simulink model "balance_leg"  (R2022b)
settings: Solver=VariableStepAuto  StartTime=0.0  StopTime=9  RelTol=1e-3
values from neighbouring files (symbols this model uses):
  K = get_K_from_LQR(R_w,R_l,l_l,l_r,l_wl,l_wr,l_bl,l_br,l_c,m_w,m_l,m_b,I_w,I_ll,I_lr,I_b,I_z,g,              R_w_ac,R_l_ac,l_l_ac,l_r_ac,l_wl_ac,l_wr_ac,l_bl_ac,l_br_ac,              l_c_ac,m_w_ac,m_l_ac,m_b_ac,I_w_ac,I_ll_ac,I_lr_ac,I_b_ac,I_z_ac,g_ac,              A,B,lqr_Q,lqr_R)    [HerKules_VOCAL_SJ_LQR_v4_with_data.m]    (also in HerKules_legth_K.m = lqr(A_num, B_num, lqr_Q, lqr_R); get_legth_k.m = lqr(JA,JB,Q,R); lqr_k.m = reshape([mt1,mt2,mt3,mt4,mt5,mt6,mt7,mt8,mt9,mt10,mt11,mt12]; niheK.m = sym('K',[2 6]))
  N = NM + mp*diff(x + L*sin(theta),t,2)    [get_legth_k.m]    (also in niheK.m)
undefined symbols (not defined in the file or in its folder): X, Y, Z
libraries: sm_lib x56, nesl_utility x22, slpidlib x2
(part 3 of 3)

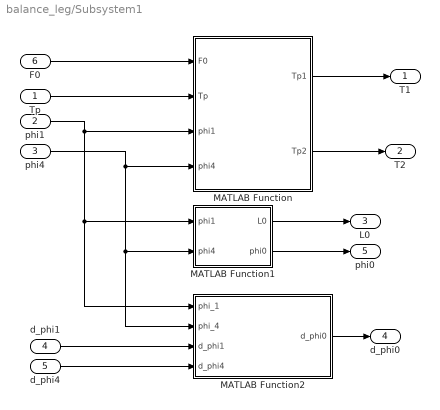
== system balance_leg/Subsystem1 ==
  Tp : Inport
  phi1 : Inport  Port=2
  phi4 : Inport  Port=3
  d_phi1 : Inport  Port=4
  d_phi4 : Inport  Port=5
  F0 : Inport  Port=6
  MATLAB Function : MATLAB Function  TreatAsAtomicUnit=on
  MATLAB Function1 : MATLAB Function  TreatAsAtomicUnit=on
  MATLAB Function2 : MATLAB Function  TreatAsAtomicUnit=on
  T1 : Outport
  T2 : Outport  Port=2
  L0 : Outport  Port=3
  d_phi0 : Outport  Port=4
  phi0 : Outport  Port=5
  wires:
  F0/1 -> MATLAB Function/1(F0)
  Tp/1 -> MATLAB Function/2(Tp)
  phi1/1 -> MATLAB Function2/1(phi_1), MATLAB Function1/1(phi1), MATLAB Function/3(phi1)
  phi4/1 -> MATLAB Function2/2(phi_4), MATLAB Function1/2(phi4), MATLAB Function/4(phi4)
  d_phi4/1 -> MATLAB Function2/4(d_phi4)
  d_phi1/1 -> MATLAB Function2/3(d_phi1)
  MATLAB Function/1(Tp1) -> T1/1
  MATLAB Function/2(Tp2) -> T2/1
  MATLAB Function1/1(L0) -> L0/1
  MATLAB Function1/2(phi0) -> phi0/1
  MATLAB Function2/1(d_phi0) -> d_phi0/1

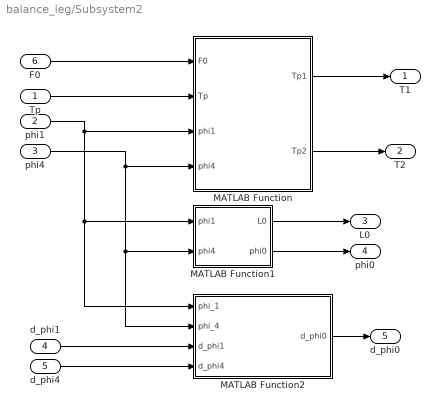
== system balance_leg/Subsystem2 ==
  Tp : Inport
  phi1 : Inport  Port=2
  phi4 : Inport  Port=3
  d_phi1 : Inport  Port=4
  d_phi4 : Inport  Port=5
  F0 : Inport  Port=6
  MATLAB Function : MATLAB Function  TreatAsAtomicUnit=on
  MATLAB Function1 : MATLAB Function  TreatAsAtomicUnit=on
  MATLAB Function2 : MATLAB Function  TreatAsAtomicUnit=on
  T1 : Outport
  T2 : Outport  Port=2
  L0 : Outport  Port=3
  phi0 : Outport  Port=4
  d_phi0 : Outport  Port=5
  wires:
  F0/1 -> MATLAB Function/1(F0)
  Tp/1 -> MATLAB Function/2(Tp)
  phi1/1 -> MATLAB Function2/1(phi_1), MATLAB Function1/1(phi1), MATLAB Function/3(phi1)
  phi4/1 -> MATLAB Function2/2(phi_4), MATLAB Function1/2(phi4), MATLAB Function/4(phi4)
  d_phi4/1 -> MATLAB Function2/4(d_phi4)
  d_phi1/1 -> MATLAB Function2/3(d_phi1)
  MATLAB Function/1(Tp1) -> T1/1
  MATLAB Function/2(Tp2) -> T2/1
  MATLAB Function1/1(L0) -> L0/1
  MATLAB Function1/2(phi0) -> phi0/1
  MATLAB Function2/1(d_phi0) -> d_phi0/1

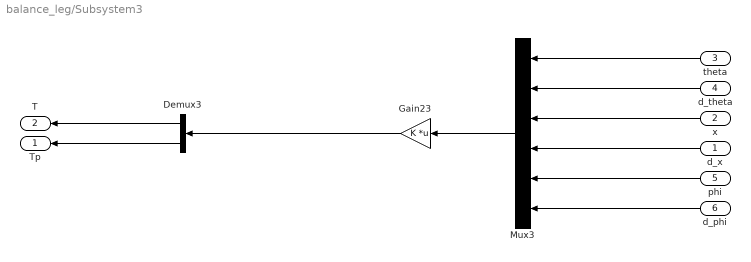
== system balance_leg/Subsystem3 ==
  d_x : Inport
  x : Inport  Port=2
  theta : Inport  Port=3
  d_theta : Inport  Port=4
  phi : Inport  Port=5
  d_phi : Inport  Port=6
  Demux3 : Demux  Outputs=2
  Gain23 : Gain  Gain=K  Multiplication=Matrix(K*u) (u vector)
  Mux3 : Mux  Inputs=6
  Tp : Outport
  T : Outport  Port=2
  wires:
  d_phi/1 -> Mux3/6
  Demux3/1 -> T/1
  d_theta/1 -> Mux3/2
  Mux3/1 -> Gain23/1
  Gain23/1 -> Demux3/1
  phi/1 -> Mux3/5
  x/1 -> Mux3/3
  theta/1 -> Mux3/1
  Demux3/2 -> Tp/1
  d_x/1 -> Mux3/4

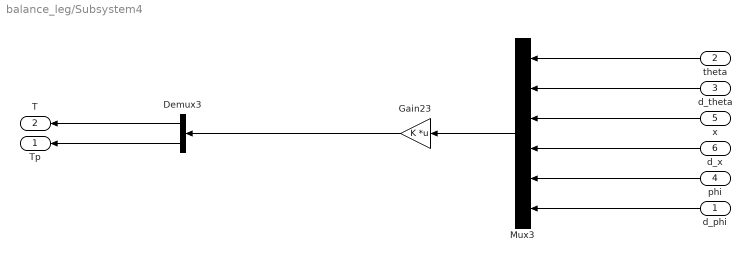
== system balance_leg/Subsystem4 ==
  d_phi : Inport
  theta : Inport  Port=2
  d_theta : Inport  Port=3
  phi : Inport  Port=4
  x : Inport  Port=5
  d_x : Inport  Port=6
  Demux3 : Demux  Outputs=2
  Gain23 : Gain  Gain=K  Multiplication=Matrix(K*u) (u vector)
  Mux3 : Mux  Inputs=6
  Tp : Outport
  T : Outport  Port=2
  wires:
  d_phi/1 -> Mux3/6
  Demux3/1 -> T/1
  d_theta/1 -> Mux3/2
  Mux3/1 -> Gain23/1
  Gain23/1 -> Demux3/1
  phi/1 -> Mux3/5
  x/1 -> Mux3/3
  theta/1 -> Mux3/1
  Demux3/2 -> Tp/1
  d_x/1 -> Mux3/4

== matlab function balance_leg/Subsystem1/MATLAB Function ==
  data: F0 input; Tp1 output; Tp input; phi1 input; phi4 input; Tp2 output
function [Tp1,Tp2] = VM_cal(F0,Tp,phi1,phi4)
% syms T1 T2 F0 Tp phi1 phi4 XE l1 l2 l3 l4
l5=0.15;
l1=0.15;
l2=0.27;
l3=0.27;
l4=0.15;

YD = l4*sin(phi4);
YB = l1*sin(phi1);
XD = l5 + l4*cos(phi4);
XB = l1*cos(phi1); 
lBD = sqrt((XD - XB)*(XD - XB) + (YD - YB)*(YD - YB));
A0 = 2*l2*(XD - XB);
B0 = 2*l2*(YD - YB);
C0 = l2*l2 + lBD*lBD - l3*l3;
phi2 = 2*atan2((B0 + sqrt(A0*A0 + B0*B0 - C0*C0)),A0 + C0);
phi3 = atan2(YB-YD+l2*sin(phi2),XB-XD+l2*cos(phi2));
XC = l1*cos(phi1) + l2*cos(phi2);
YC = l1*sin(phi1) + l2*sin(phi2);
L0 = sqrt((XC - l5/2)*(XC - l5/2) + YC*YC);
phi0 = atan2(YC,XC - l5/2);
j11 = (l1*sin(phi0-phi3)*sin(phi1-phi2))/sin(phi3-phi2);
j12 = (l1*cos(phi0-phi3)*sin(phi1-phi2))/L0*sin(phi3-phi2);
j21 = (l4*sin(phi0-phi2)*sin(phi3-phi4))/sin(phi3-phi2);
j22 = (l4*cos(phi0-phi2)*sin(phi3-phi4))/L0*sin(phi3-phi2);
J = [j11 j12; j21 j22];
F = [F0;Tp];
T = J * F;
Tp1 = T(1,1);
Tp2 = T(2,1);
end

== matlab function balance_leg/Subsystem1/MATLAB Function1 ==
  data: phi1 input; L0 output; phi4 input; phi0 output
function [L0,phi0] = get_legparam(phi1,phi4)
    l5=0.15;
    l1=0.15;
    l2=0.27;
    l3=0.27;
    l4=0.15;
    YD = l4*sin(phi4);
    YB = l1*sin(phi1);
    XD = l5 + l4*cos(phi4);
    XB = l1*cos(phi1); 
    lBD = sqrt((XD - XB)*(XD - XB) + (YD - YB)*(YD - YB));
    A0 = 2*l2*(XD - XB);
    B0 = 2*l2*(YD - YB);
    C0 = l2*l2 + lBD*lBD - l3*l3;
    phi2 = 2*atan2((B0 + sqrt(A0*A0 + B0*B0 - C0*C0)),(A0 + C0));
    XC = l1*cos(phi1) + l2*cos(phi2);
    YC = l1*sin(phi1) + l2*sin(phi2);
    L0 = sqrt((XC - l5/2)*(XC - l5/2) + YC*YC);
    phi0=atan2(YC,(XC-l5/2));
end

== matlab function balance_leg/Subsystem1/MATLAB Function2 ==
  data: phi_1 input; d_phi0 output; phi_4 input; d_phi1 input; d_phi4 input
function d_phi0 = get_dphi0(phi_1,phi_4,d_phi1,d_phi4)
    l5=0.15;
    l1=0.15;
    l2=0.27;
    l3=0.27;
    l4=0.15;
    d_phi0 = (d_phi1*((l1*cos(phi_1) + (2*l2*cos(2*atan(((4*l2^2*(l1*sin(phi_1) - l4*sin(phi_4))^2 - ((l1*sin(phi_1) - l4*sin(phi_4))^2 + (l5 - l1*cos(phi_1) + l4*cos(phi_4))^2 + l2^2 - l3^2)^2 + 4*l2^2*(l5 - l1*cos(phi_1) + l4*cos(phi_4))^2)^(1/2) - 2*l2*(l1*sin(phi_1) - l4*sin(phi_4)))/((l1*sin(phi_1) - l4*sin(phi_4))^2 + (l5 - l1*cos(phi_1) + l4*cos(phi_4))^2 + l2^2 - l3^2 + 2*l2*(l5 - l1*cos(phi_1) + l4*cos(phi_4)))))*(((8*l1*l2^2*cos(phi_1)*(l1*sin(phi_1) - l4*sin(phi_4)) - 2*(2*l1*cos(phi_1)*(l1*sin(phi_1) - l4*sin(phi_4)) + 2*l1*sin(phi_1)*(l5 - l1*cos(phi_1) + l4*cos(phi_4)))*((l1*sin(phi_1) - l4*sin(phi_4))^2 + (l5 - l1*cos(phi_1) + l4*cos(phi_4))^2 + l2^2 - l3^2) + 8*l1*l2^2*sin(phi_1)*(l5 - l1*cos(phi_1) + l4*cos(phi_4)))/(2*(4*l2^2*(l1*sin(phi_1) - l4*sin(phi_4))^2 - ((l1*sin(phi_1) - l4*sin(phi_4))^2 + (l5 - l1*cos(phi_1) + l4*cos(phi_4))^2 + l2^2 - l3^2)^2 + 4*l2^2*(l5 - l1*cos(phi_1) + l4*cos(phi_4))^2)^(1/2)) - 2*l1*l2*cos(phi_1))/((l1*sin(phi_1) - l4*sin(phi_4))^2 + (l5 - l1*cos(phi_1) + l4*cos(phi_4))^2 + l2^2 - l3^2 + 2*l2*(l5 - l1*cos(phi_1) + l4*cos(phi_4))) - (((4*l2^2*(l1*sin(phi_1) - l4*sin(phi_4))^2 - ((l1*sin(phi_1) - l4*sin(phi_4))^2 + (l5 - l1*cos(phi_1) + l4*cos(phi_4))^2 + l2^2 - l3^2)^2 + 4*l2^2*(l5 - l1*cos(phi_1) + l4*cos(phi_4))^2)^(1/2) - 2*l2*(l1*sin(phi_1) - l4*sin(phi_4)))*(2*l1*l2*sin(phi_1) + 2*l1*cos(phi_1)*(l1*sin(phi_1) - l4*sin(phi_4)) + 2*l1*sin(phi_1)*(l5 - l1*cos(phi_1) + l4*cos(phi_4))))/((l1*sin(phi_1) - l4*sin(phi_4))^2 + (l5 - l1*cos(phi_1) + l4*cos(phi_4))^2 + l2^2 - l3^2 + 2*l2*(l5 - l1*cos(phi_1) + l4*cos(phi_4)))^2))/(((4*l2^2*(l1*sin(phi_1) - l4*sin(phi_4))^2 - ((l1*sin(phi_1) - l4*sin(phi_4))^2 + (l5 - l1*cos(phi_1) + l4*cos(phi_4))^2 + l2^2 - l3^2)^2 + 4*l2^2*(l5 - l1*cos(phi_1) + l4*cos(phi_4))^2)^(1/2) - 2*l2*(l1*sin(phi_1) - l4*sin(phi_4)))^2/((l1*sin(phi_1) - l4*sin(phi_4))^2 + (l5 - l1*cos(phi_1) + l4*cos(phi_4))^2 + l2^2 - l3^2 + 2*l2*(l5 - l1*cos(phi_1) + l4*cos(phi_4)))^2 + 1))/(l2*cos(2*atan(((4*l2^2*(l1*sin(phi_1) - l4*sin(phi_4))^2 - ((l1*sin(phi_1) - l4*sin(phi_4))^2 + (l5 - l1*cos(phi_1) + l4*cos(phi_4))^2 + l2^2 - l3^2)^2 + 4*l2^2*(l5 - l1*cos(phi_1) + l4*cos(phi_4))^2)^(1/2) - 2*l2*(l1*sin(phi_1) - l4*sin(phi_4)))/((l1*sin(phi_1) - l4*sin(phi_4))^2 + (l5 - l1*cos(phi_1) + l4*cos(phi_4))^2 + l2^2 - l3^2 + 2*l2*(l5 - l1*cos(phi_1) + l4*cos(phi_4))))) - l5/2 + l1*cos(phi_1)) + ((l2*sin(2*atan(((4*l2^2*(l1*sin(phi_1) - l4*sin(phi_4))^2 - ((l1*sin(phi_1) - l4*sin(phi_4))^2 + (l5 - l1*cos(phi_1) + l4*cos(phi_4))^2 + l2^2 - l3^2)^2 + 4*l2^2*(l5 - l1*cos(phi_1) + l4*cos(phi_4))^2)^(1/2) - 2*l2*(l1*sin(phi_1) - l4*sin(phi_4)))/((l1*sin(phi_1) - l4*sin(phi_4))^2 + (l5 - l1*cos(phi_1) + l4*cos(phi_4))^2 + l2^2 - l3^2 + 2*l2*(l5 - l1*cos(phi_1) + l4*cos(phi_4))))) + l1*sin(phi_1))*(l1*sin(phi_1) + (2*l2*sin(2*atan(((4*l2^2*(l1*sin(phi_1) - l4*sin(phi_4))^2 - ((l1*sin(phi_1) - l4*sin(phi_4))^2 + (l5 - l1*cos(phi_1) + l4*cos(phi_4))^2 + l2^2 - l3^2)^2 + 4*l2^2*(l5 - l1*cos(phi_1) + l4*cos(phi_4))^2)^(1/2) - 2*l2*(l1*sin(phi_1) - l4*sin(phi_4)))/((l1*sin(phi_1) - l4*sin(phi_4))^2 + (l5 - l1*cos(phi_1) + l4*cos(phi_4))^2 + l2^2 - l3^2 + 2*l2*(l5 - l1*cos(phi_1) + l4*cos(phi_4)))))*(((8*l1*l2^2*cos(phi_1)*(l1*sin(phi_1) - l4*sin(phi_4)) - 2*(2*l1*cos(phi_1)*(l1*sin(phi_1) - l4*sin(phi_4)) + 2*l1*sin(phi_1)*(l5 - l1*cos(phi_1) + l4*cos(phi_4)))*((l1*sin(phi_1) - l4*sin(phi_4))^2 + (l5 - l1*cos(phi_1) + l4*cos(phi_4))^2 + l2^2 - l3^2) + 8*l1*l2^2*sin(phi_1)*(l5 - l1*cos(phi_1) + l4*cos(phi_4)))/(2*(4*l2^2*(l1*sin(phi_1) - l4*sin(phi_4))^2 - ((l1*sin(phi_1) - l4*sin(phi_4))^2 + (l5 - l1*cos(phi_1) + l4*cos(phi_4))^2 + l2^2 - l3^2)^2 + 4*l2^2*(l5 - l1*cos(phi_1) + l4*cos(phi_4))^2)^(1/2)) - 2*l1*l2*cos(phi_1))/((l1*sin(phi_1) - l4*sin(phi_4))^2 + (l5 - l1*cos(phi_1) + l4*cos(phi_4))^2 + l2^2 - l3^2 + 2*l2*(l5 - l1*cos(phi_1) + l4*cos(phi_4))) - (((4*l2^2*(l1*sin(phi_1) - l4*sin(phi_4))^2 - ((l1*sin(phi_1) - l4*sin(phi_4))^2 + (l5 - l1*cos(phi_1) + l4*cos(phi_4))^2 + l2^2 - l3^2)^2 + 4*l2^2*(l5 - l1*cos(phi_1) + l4*cos(phi_4))^2)^(1/2) - 2*l2*(l1*sin(phi_1) - l4*sin(phi_4)))*(2*l1*l2*sin(phi_1) + 2*l1*cos(phi_1)*(l1*sin(phi_1) - l4*sin(phi_4)) + 2*l1*sin(phi_1)*(l5 - l1*cos(phi_1) + l4*cos(phi_4))))/((l1*sin(phi_1) - l4*sin(phi_4))^2 + (l5 - l1*cos(phi_1) + l4*cos(phi_4))^2 + l2^2 - l3^2 + 2*l2*(l5 - l1*cos(phi_1) + l4*cos(phi_4)))^2))/(((4*l2^2*(l1*sin(phi_1) - l4*sin(phi_4))^2 - ((l1*sin(phi_1) - l4*sin(phi_4))^2 + (l5 - l1*cos(phi_1) + l4*cos(phi_4))^2 + l2^2 - l3^2)^2 + 4*l2^2*(l5 - l1*cos(phi_1) + l4*cos(phi_4))^2)^(1/2) - 2*l2*(l1*sin(phi_1) - l4*sin(phi_4)))^2/((l1*sin(phi_1) - l4*sin(phi_4))^2 + (l5 - l1*cos(phi_1) + l4*cos(phi_4))^2 + l2^2 - l3^2 + 2*l2*(l5 - l1*cos(phi_1) + l4*cos(phi_4)))^2 + 1)))/(l2*cos(2*atan(((4*l2^2*(l1*sin(phi_1) - l4*sin(phi_4))^2 - ((l1*sin(phi_1) - l4*sin(phi_4))^2 + (l5 - l1*cos(phi_1) + l4*cos(phi_4))^2 + l2^2 - l3^2)^2 + 4*l2^2*(l5 - l1*cos(phi_1) + l4*cos(phi_4))^2)^(1/2) - 2*l2*(l1*sin(phi_1) - l4*sin(phi_4)))/((l1*sin(phi_1) - l4*sin(phi_4))^2 + (l5 - l1*cos(phi_1) + l4*cos(phi_4))^2 + l2^2 - l3^2 + 2*l2*(l5 - l1*cos(phi_1) + l4*cos(phi_4))))) - l5/2 + l1*cos(phi_1))^2))/((l2*sin(2*atan(((4*l2^2*(l1*sin(phi_1) - l4*sin(phi_4))^2 - ((l1*sin(phi_1) - l4*sin(phi_4))^2 + (l5 - l1*cos(phi_1) + l4*cos(phi_4))^2 + l2^2 - l3^2)^2 + 4*l2^2*(l5 - l1*cos(phi_1) + l4*cos(phi_4))^2)^(1/2) - 2*l2*(l1*sin(phi_1) - l4*sin(phi_4)))/((l1*sin(phi_1) - l4*sin(phi_4))^2 + (l5 - l1*cos(phi_1) + l4*cos(phi_4))^2 + l2^2 - l3^2 + 2*l2*(l5 - l1*cos(phi_1) + l4*cos(phi_4))))) + l1*sin(phi_1))^2/(l2*cos(2*atan(((4*l2^2*(l1*sin(phi_1) - l4*sin(phi_4))^2 - ((l1*sin(phi_1) - l4*sin(phi_4))^2 + (l5 - l1*cos(phi_1) + l4*cos(phi_4))^2 + l2^2 - l3^2)^2 + 4*l2^2*(l5 - l1*cos(phi_1) + l4*cos(phi_4))^2)^(1/2) - 2*l2*(l1*sin(phi_1) - l4*sin(phi_4)))/((l1*sin(phi_1) - l4*sin(phi_4))^2 + (l5 - l1*cos(phi_1) + l4*cos(phi_4))^2 + l2^2 - l3^2 + 2*l2*(l5 - l1*cos(phi_1) + l4*cos(phi_4))))) - l5/2 + l1*cos(phi_1))^2 + 1) - (d_phi4*((2*l2*cos(2*atan(((4*l2^2*(l1*sin(phi_1) - l4*sin(phi_4))^2 - ((l1*sin(phi_1) - l4*sin(phi_4))^2 + (l5 - l1*cos(phi_1) + l4*cos(phi_4))^2 + l2^2 - l3^2)^2 + 4*l2^2*(l5 - l1*cos(phi_1) + l4*cos(phi_4))^2)^(1/2) - 2*l2*(l1*sin(phi_1) - l4*sin(phi_4)))/((l1*sin(phi_1) - l4*sin(phi_4))^2 + (l5 - l1*cos(phi_1) + l4*cos(phi_4))^2 + l2^2 - l3^2 + 2*l2*(l5 - l1*cos(phi_1) + l4*cos(phi_4)))))*(((8*l2^2*l4*cos(phi_4)*(l1*sin(phi_1) - l4*sin(phi_4)) - 2*(2*l4*cos(phi_4)*(l1*sin(phi_1) - l4*sin(phi_4)) + 2*l4*sin(phi_4)*(l5 - l1*cos(phi_1) + l4*cos(phi_4)))*((l1*sin(phi_1) - l4*sin(phi_4))^2 + (l5 - l1*cos(phi_1) + l4*cos(phi_4))^2 + l2^2 - l3^2) + 8*l2^2*l4*sin(phi_4)*(l5 - l1*cos(phi_1) + l4*cos(phi_4)))/(2*(4*l2^2*(l1*sin(phi_1) - l4*sin(phi_4))^2 - ((l1*sin(phi_1) - l4*sin(phi_4))^2 + (l5 - l1*cos(phi_1) + l4*cos(phi_4))^2 + l2^2 - l3^2)^2 + 4*l2^2*(l5 - l1*cos(phi_1) + l4*cos(phi_4))^2)^(1/2)) - 2*l2*l4*cos(phi_4))/((l1*sin(phi_1) - l4*sin(phi_4))^2 + (l5 - l1*cos(phi_1) + l4*cos(phi_4))^2 + l2^2 - l3^2 + 2*l2*(l5 - l1*cos(phi_1) + l4*cos(phi_4))) - (((4*l2^2*(l1*sin(phi_1) - l4*sin(phi_4))^2 - ((l1*sin(phi_1) - l4*sin(phi_4))^2 + (l5 - l1*cos(phi_1) + l4*cos(phi_4))^2 + l2^2 - l3^2)^2 + 4*l2^2*(l5 - l1*cos(phi_1) + l4*cos(phi_4))^2)^(1/2) - 2*l2*(l1*sin(phi_1) - l4*sin(phi_4)))*(2*l2*l4*sin(phi_4) + 2*l4*cos(phi_4)*(l1*sin(phi_1) - l4*sin(phi_4)) + 2*l4*sin(phi_4)*(l5 - l1*cos(phi_1) + l4*cos(phi_4))))/((l1*sin(phi_1) - l4*sin(phi_4))^2 + (l5 - l1*cos(phi_1) + l4*cos(phi_4))^2 + l2^2 - l3^2 + 2*l2*(l5 - l1*cos(phi_1) + l4*cos(phi_4)))^2))/((((4*l2^2*(l1*sin(phi_1) - l4*sin(phi_4))^2 - ((l1*sin(phi_1) - l4*sin(phi_4))^2 + (l5 - l1*cos(phi_1) + l4*cos(phi_4))^2 + l2^2 - l3^2)^2 + 4*l2^2*(l5 - l1*cos(phi_1) + l4*cos(phi_4))^2)^(1/2) - 2*l2*(l1*sin(phi_1) - l4*sin(phi_4)))^2/((l1*sin(phi_1) - l4*sin(phi_4))^2 + (l5 - l1*cos(phi_1) + l4*cos(phi_4))^2 + l2^2 - l3^2 + 2*l2*(l5 - l1*cos(phi_1) + l4*cos(phi_4)))^2 + 1)*(l2*cos(2*atan(((4*l2^2*(l1*sin(phi_1) - l4*sin(phi_4))^2 - ((l1*sin(phi_1) - l4*sin(phi_4))^2 + (l5 - l1*cos(phi_1) + l4*cos(phi_4))^2 + l2^2 - l3^2)^2 + 4*l2^2*(l5 - l1*cos(phi_1) + l4*cos(phi_4))^2)^(1/2) - 2*l2*(l1*sin(phi_1) - l4*sin(phi_4)))/((l1*sin(phi_1) - l4*sin(phi_4))^2 + (l5 - l1*cos(phi_1) + l4*cos(phi_4))^2 + l2^2 - l3^2 + 2*l2*(l5 - l1*cos(phi_1) + l4*cos(phi_4))))) - l5/2 + l1*cos(phi_1))) + (2*l2*sin(2*atan(((4*l2^2*(l1*sin(phi_1) - l4*sin(phi_4))^2 - ((l1*sin(phi_1) - l4*sin(phi_4))^2 + (l5 - l1*cos(phi_1) + l4*cos(phi_4))^2 + l2^2 - l3^2)^2 + 4*l2^2*(l5 - l1*cos(phi_1) + l4*cos(phi_4))^2)^(1/2) - 2*l2*(l1*sin(phi_1) - l4*sin(phi_4)))/((l1*sin(phi_1) - l4*sin(phi_4))^2 + (l5 - l1*cos(phi_1) + l4*cos(phi_4))^2 + l2^2 - l3^2 + 2*l2*(l5 - l1*cos(phi_1) + l4*cos(phi_4)))))*(l2*sin(2*atan(((4*l2^2*(l1*sin(phi_1) - l4*sin(phi_4))^2 - ((l1*sin(phi_1) - l4*sin(phi_4))^2 + (l5 - l1*cos(phi_1) + l4*cos(phi_4))^2 + l2^2 - l3^2)^2 + 4*l2^2*(l5 - l1*cos(phi_1) + l4*cos(phi_4))^2)^(1/2) - 2*l2*(l1*sin(phi_1) - l4*sin(phi_4)))/((l1*sin(phi_1) - l4*sin(phi_4))^2 + (l5 - l1*cos(phi_1) + l4*cos(phi_4))^2 + l2^2 - l3^2 + 2*l2*(l5 - l1*cos(phi_1) + l4*cos(phi_4))))) + l1*sin(phi_1))*(((8*l2^2*l4*cos(phi_4)*(l1*sin(phi_1) - l4*sin(phi_4)) - 2*(2*l4*cos(phi_4)*(l1*sin(phi_1) - l4*sin(phi_4)) + 2*l4*sin(phi_4)*(l5 - l1*cos(phi_1) + l4*cos(phi_4)))*((l1*sin(phi_1) - l4*sin(phi_4))^2 + (l5 - l1*cos(phi_1) + l4*cos(phi_4))^2 + l2^2 - l3^2) + 8*l2^2*l4*sin(phi_4)*(l5 - l1*cos(phi_1) + l4*cos(phi_4)))/(2*(4*l2^2*(l1*sin(phi_1) - l4*sin(phi_4))^2 - ((l1*sin(phi_1) - l4*sin(phi_4))^2 + (l5 - l1*cos(phi_1) + l4*cos(phi_4))^2 + l2^2 - l3^2)^2 + 4*l2^2*(l5 - l1*cos(phi_1) + l4*cos(phi_4))^2)^(1/2)) - 2*l2*l4*cos(phi_4))/((l1*sin(phi_1) - l4*sin(phi_4))^2 + (l5 - l1*cos(phi_1) + l4*cos(phi_4))^2 + l2^2 - l3^2 + 2*l2*(l5 - l1*cos(phi_1) + l4*cos(phi_4))) - (((4*l2^2*(l1*sin(phi_1) - l4*sin(phi_4))^2 - ((l1*sin(phi_1) - l4*sin(phi_4))^2 + (l5 - l1*cos(phi_1) + l4*cos(phi_4))^2 + l2^2 - l3^2)^2 + 4*l2^2*(l5 - l1*cos(phi_1) + l4*cos(phi_4))^2)^(1/2) - 2*l2*(l1*sin(phi_1) - l4*sin(phi_4)))*(2*l2*l4*sin(phi_4) + 2*l4*cos(phi_4)*(l1*sin(phi_1) - l4*sin(phi_4)) + 2*l4*sin(phi_4)*(l5 - l1*cos(phi_1) + l4*cos(phi_4))))/((l1*sin(phi_1) - l4*sin(phi_4))^2 + (l5 - l1*cos(phi_1) + l4*cos(phi_4))^2 + l2^2 - l3^2 + 2*l2*(l5 - l1*cos(phi_1) + l4*cos(phi_4)))^2))/((((4*l2^2*(l1*sin(phi_1) - l4*sin(phi_4))^2 - ((l1*sin(phi_1) - l4*sin(phi_4))^2 + (l5 - l1*cos(phi_1) + l4*cos(phi_4))^2 + l2^2 - l3^2)^2 + 4*l2^2*(l5 - l1*cos(phi_1) + l4*cos(phi_4))^2)^(1/2) - 2*l2*(l1*sin(phi_1) - l4*sin(phi_4)))^2/((l1*sin(phi_1) - l4*sin(phi_4))^2 + (l5 - l1*cos(phi_1) + l4*cos(phi_4))^2 + l2^2 - l3^2 + 2*l2*(l5 - l1*cos(phi_1) + l4*cos(phi_4)))^2 + 1)*(l2*cos(2*atan(((4*l2^2*(l1*sin(phi_1) - l4*sin(phi_4))^2 - ((l1*sin(phi_1) - l4*sin(phi_4))^2 + (l5 - l1*cos(phi_1) + l4*cos(phi_4))^2 + l2^2 - l3^2)^2 + 4*l2^2*(l5 - l1*cos(phi_1) + l4*cos(phi_4))^2)^(1/2) - 2*l2*(l1*sin(phi_1) - l4*sin(phi_4)))/((l1*sin(phi_1) - l4*sin(phi_4))^2 + (l5 - l1*cos(phi_1) + l4*cos(phi_4))^2 + l2^2 - l3^2 + 2*l2*(l5 - l1*cos(phi_1) + l4*cos(phi_4))))) - l5/2 + l1*cos(phi_1))^2)))/((l2*sin(2*atan(((4*l2^2*(l1*sin(phi_1) - l4*sin(phi_4))^2 - ((l1*sin(phi_1) - l4*sin(phi_4))^2 + (l5 - l1*cos(phi_1) + l4*cos(phi_4))^2 + l2^2 - l3^2)^2 + 4*l2^2*(l5 - l1*cos(phi_1) + l4*cos(phi_4))^2)^(1/2) - 2*l2*(l1*sin(phi_1) - l4*sin(phi_4)))/((l1*sin(phi_1) - l4*sin(phi_4))^2 + (l5 - l1*cos(phi_1) + l4*cos(phi_4))^2 + l2^2 - l3^2 + 2*l2*(l5 - l1*cos(phi_1) + l4*cos(phi_4))))) + l1*sin(phi_1))^2/(l2*cos(2*atan(((4*l2^2*(l1*sin(phi_1) - l4*sin(phi_4))^2 - ((l1*sin(phi_1) - l4*sin(phi_4))^2 + (l5 - l1*cos(phi_1) + l4*cos(phi_4))^2 + l2^2 - l3^2)^2 + 4*l2^2*(l5 - l1*cos(phi_1) + l4*cos(phi_4))^2)^(1/2) - 2*l2*(l1*sin(phi_1) - l4*sin(phi_4)))/((l1*sin(phi_1) - l4*sin(phi_4))^2 + (l5 - l1*cos(phi_1) + l4*cos(phi_4))^2 + l2^2 - l3^2 + 2*l2*(l5 - l1*cos(phi_1) + l4*cos(phi_4))))) - l5/2 + l1*cos(phi_1))^2 + 1);
end

== matlab function balance_leg/Subsystem2/MATLAB Function ==
  data: F0 input; Tp1 output; Tp input; phi1 input; phi4 input; Tp2 output
function [Tp1,Tp2] = VM_cal(F0,Tp,phi1,phi4)
% syms T1 T2 F0 Tp phi1 phi4 XE l1 l2 l3 l4
l5=0.15;
l1=0.15;
l2=0.27;
l3=0.27;
l4=0.15;

YD = l4*sin(phi4);
YB = l1*sin(phi1);
XD = l5 + l4*cos(phi4);
XB = l1*cos(phi1); 
lBD = sqrt((XD - XB)*(XD - XB) + (YD - YB)*(YD - YB));
A0 = 2*l2*(XD - XB);
B0 = 2*l2*(YD - YB);
C0 = l2*l2 + lBD*lBD - l3*l3;
phi2 = 2*atan2((B0 + sqrt(A0*A0 + B0*B0 - C0*C0)),A0 + C0);
phi3 = atan2(YB-YD+l2*sin(phi2),XB-XD+l2*cos(phi2));
XC = l1*cos(phi1) + l2*cos(phi2);
YC = l1*sin(phi1) + l2*sin(phi2);
L0 = sqrt((XC - l5/2)*(XC - l5/2) + YC*YC);
phi0 = atan2(YC,XC - l5/2);
j11 = (l1*sin(phi0-phi3)*sin(phi1-phi2))/sin(phi3-phi2);
j12 = (l1*cos(phi0-phi3)*sin(phi1-phi2))/L0*sin(phi3-phi2);
j21 = (l4*sin(phi0-phi2)*sin(phi3-phi4))/sin(phi3-phi2);
j22 = (l4*cos(phi0-phi2)*sin(phi3-phi4))/L0*sin(phi3-phi2);
J = [j11 j12; j21 j22];
F = [F0;Tp];
T = J * F;
Tp1 = T(1,1);
Tp2 = T(2,1);
end

== matlab function balance_leg/Subsystem2/MATLAB Function1 ==
  data: phi1 input; L0 output; phi4 input; phi0 output
function [L0,phi0] = get_legparam(phi1,phi4)
    l5=0.15;
    l1=0.15;
    l2=0.27;
    l3=0.27;
    l4=0.15;
    YD = l4*sin(phi4);
    YB = l1*sin(phi1);
    XD = l5 + l4*cos(phi4);
    XB = l1*cos(phi1); 
    lBD = sqrt((XD - XB)*(XD - XB) + (YD - YB)*(YD - YB));
    A0 = 2*l2*(XD - XB);
    B0 = 2*l2*(YD - YB);
    C0 = l2*l2 + lBD*lBD - l3*l3;
    phi2 = 2*atan2((B0 + sqrt(A0*A0 + B0*B0 - C0*C0)),(A0 + C0));
    XC = l1*cos(phi1) + l2*cos(phi2);
    YC = l1*sin(phi1) + l2*sin(phi2);
    L0 = sqrt((XC - l5/2)*(XC - l5/2) + YC*YC);
    phi0=atan2(YC,(XC-l5/2));
end

== matlab function balance_leg/Subsystem2/MATLAB Function2 ==
  data: phi_1 input; d_phi0 output; phi_4 input; d_phi1 input; d_phi4 input
function d_phi0 = get_dphi0(phi_1,phi_4,d_phi1,d_phi4)
    l5=0.15;
    l1=0.15;
    l2=0.27;
    l3=0.27;
    l4=0.15;
    d_phi0 = (d_phi1*((l1*cos(phi_1) + (2*l2*cos(2*atan(((4*l2^2*(l1*sin(phi_1) - l4*sin(phi_4))^2 - ((l1*sin(phi_1) - l4*sin(phi_4))^2 + (l5 - l1*cos(phi_1) + l4*cos(phi_4))^2 + l2^2 - l3^2)^2 + 4*l2^2*(l5 - l1*cos(phi_1) + l4*cos(phi_4))^2)^(1/2) - 2*l2*(l1*sin(phi_1) - l4*sin(phi_4)))/((l1*sin(phi_1) - l4*sin(phi_4))^2 + (l5 - l1*cos(phi_1) + l4*cos(phi_4))^2 + l2^2 - l3^2 + 2*l2*(l5 - l1*cos(phi_1) + l4*cos(phi_4)))))*(((8*l1*l2^2*cos(phi_1)*(l1*sin(phi_1) - l4*sin(phi_4)) - 2*(2*l1*cos(phi_1)*(l1*sin(phi_1) - l4*sin(phi_4)) + 2*l1*sin(phi_1)*(l5 - l1*cos(phi_1) + l4*cos(phi_4)))*((l1*sin(phi_1) - l4*sin(phi_4))^2 + (l5 - l1*cos(phi_1) + l4*cos(phi_4))^2 + l2^2 - l3^2) + 8*l1*l2^2*sin(phi_1)*(l5 - l1*cos(phi_1) + l4*cos(phi_4)))/(2*(4*l2^2*(l1*sin(phi_1) - l4*sin(phi_4))^2 - ((l1*sin(phi_1) - l4*sin(phi_4))^2 + (l5 - l1*cos(phi_1) + l4*cos(phi_4))^2 + l2^2 - l3^2)^2 + 4*l2^2*(l5 - l1*cos(phi_1) + l4*cos(phi_4))^2)^(1/2)) - 2*l1*l2*cos(phi_1))/((l1*sin(phi_1) - l4*sin(phi_4))^2 + (l5 - l1*cos(phi_1) + l4*cos(phi_4))^2 + l2^2 - l3^2 + 2*l2*(l5 - l1*cos(phi_1) + l4*cos(phi_4))) - (((4*l2^2*(l1*sin(phi_1) - l4*sin(phi_4))^2 - ((l1*sin(phi_1) - l4*sin(phi_4))^2 + (l5 - l1*cos(phi_1) + l4*cos(phi_4))^2 + l2^2 - l3^2)^2 + 4*l2^2*(l5 - l1*cos(phi_1) + l4*cos(phi_4))^2)^(1/2) - 2*l2*(l1*sin(phi_1) - l4*sin(phi_4)))*(2*l1*l2*sin(phi_1) + 2*l1*cos(phi_1)*(l1*sin(phi_1) - l4*sin(phi_4)) + 2*l1*sin(phi_1)*(l5 - l1*cos(phi_1) + l4*cos(phi_4))))/((l1*sin(phi_1) - l4*sin(phi_4))^2 + (l5 - l1*cos(phi_1) + l4*cos(phi_4))^2 + l2^2 - l3^2 + 2*l2*(l5 - l1*cos(phi_1) + l4*cos(phi_4)))^2))/(((4*l2^2*(l1*sin(phi_1) - l4*sin(phi_4))^2 - ((l1*sin(phi_1) - l4*sin(phi_4))^2 + (l5 - l1*cos(phi_1) + l4*cos(phi_4))^2 + l2^2 - l3^2)^2 + 4*l2^2*(l5 - l1*cos(phi_1) + l4*cos(phi_4))^2)^(1/2) - 2*l2*(l1*sin(phi_1) - l4*sin(phi_4)))^2/((l1*sin(phi_1) - l4*sin(phi_4))^2 + (l5 - l1*cos(phi_1) + l4*cos(phi_4))^2 + l2^2 - l3^2 + 2*l2*(l5 - l1*cos(phi_1) + l4*cos(phi_4)))^2 + 1))/(l2*cos(2*atan(((4*l2^2*(l1*sin(phi_1) - l4*sin(phi_4))^2 - ((l1*sin(phi_1) - l4*sin(phi_4))^2 + (l5 - l1*cos(phi_1) + l4*cos(phi_4))^2 + l2^2 - l3^2)^2 + 4*l2^2*(l5 - l1*cos(phi_1) + l4*cos(phi_4))^2)^(1/2) - 2*l2*(l1*sin(phi_1) - l4*sin(phi_4)))/((l1*sin(phi_1) - l4*sin(phi_4))^2 + (l5 - l1*cos(phi_1) + l4*cos(phi_4))^2 + l2^2 - l3^2 + 2*l2*(l5 - l1*cos(phi_1) + l4*cos(phi_4))))) - l5/2 + l1*cos(phi_1)) + ((l2*sin(2*atan(((4*l2^2*(l1*sin(phi_1) - l4*sin(phi_4))^2 - ((l1*sin(phi_1) - l4*sin(phi_4))^2 + (l5 - l1*cos(phi_1) + l4*cos(phi_4))^2 + l2^2 - l3^2)^2 + 4*l2^2*(l5 - l1*cos(phi_1) + l4*cos(phi_4))^2)^(1/2) - 2*l2*(l1*sin(phi_1) - l4*sin(phi_4)))/((l1*sin(phi_1) - l4*sin(phi_4))^2 + (l5 - l1*cos(phi_1) + l4*cos(phi_4))^2 + l2^2 - l3^2 + 2*l2*(l5 - l1*cos(phi_1) + l4*cos(phi_4))))) + l1*sin(phi_1))*(l1*sin(phi_1) + (2*l2*sin(2*atan(((4*l2^2*(l1*sin(phi_1) - l4*sin(phi_4))^2 - ((l1*sin(phi_1) - l4*sin(phi_4))^2 + (l5 - l1*cos(phi_1) + l4*cos(phi_4))^2 + l2^2 - l3^2)^2 + 4*l2^2*(l5 - l1*cos(phi_1) + l4*cos(phi_4))^2)^(1/2) - 2*l2*(l1*sin(phi_1) - l4*sin(phi_4)))/((l1*sin(phi_1) - l4*sin(phi_4))^2 + (l5 - l1*cos(phi_1) + l4*cos(phi_4))^2 + l2^2 - l3^2 + 2*l2*(l5 - l1*cos(phi_1) + l4*cos(phi_4)))))*(((8*l1*l2^2*cos(phi_1)*(l1*sin(phi_1) - l4*sin(phi_4)) - 2*(2*l1*cos(phi_1)*(l1*sin(phi_1) - l4*sin(phi_4)) + 2*l1*sin(phi_1)*(l5 - l1*cos(phi_1) + l4*cos(phi_4)))*((l1*sin(phi_1) - l4*sin(phi_4))^2 + (l5 - l1*cos(phi_1) + l4*cos(phi_4))^2 + l2^2 - l3^2) + 8*l1*l2^2*sin(phi_1)*(l5 - l1*cos(phi_1) + l4*cos(phi_4)))/(2*(4*l2^2*(l1*sin(phi_1) - l4*sin(phi_4))^2 - ((l1*sin(phi_1) - l4*sin(phi_4))^2 + (l5 - l1*cos(phi_1) + l4*cos(phi_4))^2 + l2^2 - l3^2)^2 + 4*l2^2*(l5 - l1*cos(phi_1) + l4*cos(phi_4))^2)^(1/2)) - 2*l1*l2*cos(phi_1))/((l1*sin(phi_1) - l4*sin(phi_4))^2 + (l5 - l1*cos(phi_1) + l4*cos(phi_4))^2 + l2^2 - l3^2 + 2*l2*(l5 - l1*cos(phi_1) + l4*cos(phi_4))) - (((4*l2^2*(l1*sin(phi_1) - l4*sin(phi_4))^2 - ((l1*sin(phi_1) - l4*sin(phi_4))^2 + (l5 - l1*cos(phi_1) + l4*cos(phi_4))^2 + l2^2 - l3^2)^2 + 4*l2^2*(l5 - l1*cos(phi_1) + l4*cos(phi_4))^2)^(1/2) - 2*l2*(l1*sin(phi_1) - l4*sin(phi_4)))*(2*l1*l2*sin(phi_1) + 2*l1*cos(phi_1)*(l1*sin(phi_1) - l4*sin(phi_4)) + 2*l1*sin(phi_1)*(l5 - l1*cos(phi_1) + l4*cos(phi_4))))/((l1*sin(phi_1) - l4*sin(phi_4))^2 + (l5 - l1*cos(phi_1) + l4*cos(phi_4))^2 + l2^2 - l3^2 + 2*l2*(l5 - l1*cos(phi_1) + l4*cos(phi_4)))^2))/(((4*l2^2*(l1*sin(phi_1) - l4*sin(phi_4))^2 - ((l1*sin(phi_1) - l4*sin(phi_4))^2 + (l5 - l1*cos(phi_1) + l4*cos(phi_4))^2 + l2^2 - l3^2)^2 + 4*l2^2*(l5 - l1*cos(phi_1) + l4*cos(phi_4))^2)^(1/2) - 2*l2*(l1*sin(phi_1) - l4*sin(phi_4)))^2/((l1*sin(phi_1) - l4*sin(phi_4))^2 + (l5 - l1*cos(phi_1) + l4*cos(phi_4))^2 + l2^2 - l3^2 + 2*l2*(l5 - l1*cos(phi_1) + l4*cos(phi_4)))^2 + 1)))/(l2*cos(2*atan(((4*l2^2*(l1*sin(phi_1) - l4*sin(phi_4))^2 - ((l1*sin(phi_1) - l4*sin(phi_4))^2 + (l5 - l1*cos(phi_1) + l4*cos(phi_4))^2 + l2^2 - l3^2)^2 + 4*l2^2*(l5 - l1*cos(phi_1) + l4*cos(phi_4))^2)^(1/2) - 2*l2*(l1*sin(phi_1) - l4*sin(phi_4)))/((l1*sin(phi_1) - l4*sin(phi_4))^2 + (l5 - l1*cos(phi_1) + l4*cos(phi_4))^2 + l2^2 - l3^2 + 2*l2*(l5 - l1*cos(phi_1) + l4*cos(phi_4))))) - l5/2 + l1*cos(phi_1))^2))/((l2*sin(2*atan(((4*l2^2*(l1*sin(phi_1) - l4*sin(phi_4))^2 - ((l1*sin(phi_1) - l4*sin(phi_4))^2 + (l5 - l1*cos(phi_1) + l4*cos(phi_4))^2 + l2^2 - l3^2)^2 + 4*l2^2*(l5 - l1*cos(phi_1) + l4*cos(phi_4))^2)^(1/2) - 2*l2*(l1*sin(phi_1) - l4*sin(phi_4)))/((l1*sin(phi_1) - l4*sin(phi_4))^2 + (l5 - l1*cos(phi_1) + l4*cos(phi_4))^2 + l2^2 - l3^2 + 2*l2*(l5 - l1*cos(phi_1) + l4*cos(phi_4))))) + l1*sin(phi_1))^2/(l2*cos(2*atan(((4*l2^2*(l1*sin(phi_1) - l4*sin(phi_4))^2 - ((l1*sin(phi_1) - l4*sin(phi_4))^2 + (l5 - l1*cos(phi_1) + l4*cos(phi_4))^2 + l2^2 - l3^2)^2 + 4*l2^2*(l5 - l1*cos(phi_1) + l4*cos(phi_4))^2)^(1/2) - 2*l2*(l1*sin(phi_1) - l4*sin(phi_4)))/((l1*sin(phi_1) - l4*sin(phi_4))^2 + (l5 - l1*cos(phi_1) + l4*cos(phi_4))^2 + l2^2 - l3^2 + 2*l2*(l5 - l1*cos(phi_1) + l4*cos(phi_4))))) - l5/2 + l1*cos(phi_1))^2 + 1) - (d_phi4*((2*l2*cos(2*atan(((4*l2^2*(l1*sin(phi_1) - l4*sin(phi_4))^2 - ((l1*sin(phi_1) - l4*sin(phi_4))^2 + (l5 - l1*cos(phi_1) + l4*cos(phi_4))^2 + l2^2 - l3^2)^2 + 4*l2^2*(l5 - l1*cos(phi_1) + l4*cos(phi_4))^2)^(1/2) - 2*l2*(l1*sin(phi_1) - l4*sin(phi_4)))/((l1*sin(phi_1) - l4*sin(phi_4))^2 + (l5 - l1*cos(phi_1) + l4*cos(phi_4))^2 + l2^2 - l3^2 + 2*l2*(l5 - l1*cos(phi_1) + l4*cos(phi_4)))))*(((8*l2^2*l4*cos(phi_4)*(l1*sin(phi_1) - l4*sin(phi_4)) - 2*(2*l4*cos(phi_4)*(l1*sin(phi_1) - l4*sin(phi_4)) + 2*l4*sin(phi_4)*(l5 - l1*cos(phi_1) + l4*cos(phi_4)))*((l1*sin(phi_1) - l4*sin(phi_4))^2 + (l5 - l1*cos(phi_1) + l4*cos(phi_4))^2 + l2^2 - l3^2) + 8*l2^2*l4*sin(phi_4)*(l5 - l1*cos(phi_1) + l4*cos(phi_4)))/(2*(4*l2^2*(l1*sin(phi_1) - l4*sin(phi_4))^2 - ((l1*sin(phi_1) - l4*sin(phi_4))^2 + (l5 - l1*cos(phi_1) + l4*cos(phi_4))^2 + l2^2 - l3^2)^2 + 4*l2^2*(l5 - l1*cos(phi_1) + l4*cos(phi_4))^2)^(1/2)) - 2*l2*l4*cos(phi_4))/((l1*sin(phi_1) - l4*sin(phi_4))^2 + (l5 - l1*cos(phi_1) + l4*cos(phi_4))^2 + l2^2 - l3^2 + 2*l2*(l5 - l1*cos(phi_1) + l4*cos(phi_4))) - (((4*l2^2*(l1*sin(phi_1) - l4*sin(phi_4))^2 - ((l1*sin(phi_1) - l4*sin(phi_4))^2 + (l5 - l1*cos(phi_1) + l4*cos(phi_4))^2 + l2^2 - l3^2)^2 + 4*l2^2*(l5 - l1*cos(phi_1) + l4*cos(phi_4))^2)^(1/2) - 2*l2*(l1*sin(phi_1) - l4*sin(phi_4)))*(2*l2*l4*sin(phi_4) + 2*l4*cos(phi_4)*(l1*sin(phi_1) - l4*sin(phi_4)) + 2*l4*sin(phi_4)*(l5 - l1*cos(phi_1) + l4*cos(phi_4))))/((l1*sin(phi_1) - l4*sin(phi_4))^2 + (l5 - l1*cos(phi_1) + l4*cos(phi_4))^2 + l2^2 - l3^2 + 2*l2*(l5 - l1*cos(phi_1) + l4*cos(phi_4)))^2))/((((4*l2^2*(l1*sin(phi_1) - l4*sin(phi_4))^2 - ((l1*sin(phi_1) - l4*sin(phi_4))^2 + (l5 - l1*cos(phi_1) + l4*cos(phi_4))^2 + l2^2 - l3^2)^2 + 4*l2^2*(l5 - l1*cos(phi_1) + l4*cos(phi_4))^2)^(1/2) - 2*l2*(l1*sin(phi_1) - l4*sin(phi_4)))^2/((l1*sin(phi_1) - l4*sin(phi_4))^2 + (l5 - l1*cos(phi_1) + l4*cos(phi_4))^2 + l2^2 - l3^2 + 2*l2*(l5 - l1*cos(phi_1) + l4*cos(phi_4)))^2 + 1)*(l2*cos(2*atan(((4*l2^2*(l1*sin(phi_1) - l4*sin(phi_4))^2 - ((l1*sin(phi_1) - l4*sin(phi_4))^2 + (l5 - l1*cos(phi_1) + l4*cos(phi_4))^2 + l2^2 - l3^2)^2 + 4*l2^2*(l5 - l1*cos(phi_1) + l4*cos(phi_4))^2)^(1/2) - 2*l2*(l1*sin(phi_1) - l4*sin(phi_4)))/((l1*sin(phi_1) - l4*sin(phi_4))^2 + (l5 - l1*cos(phi_1) + l4*cos(phi_4))^2 + l2^2 - l3^2 + 2*l2*(l5 - l1*cos(phi_1) + l4*cos(phi_4))))) - l5/2 + l1*cos(phi_1))) + (2*l2*sin(2*atan(((4*l2^2*(l1*sin(phi_1) - l4*sin(phi_4))^2 - ((l1*sin(phi_1) - l4*sin(phi_4))^2 + (l5 - l1*cos(phi_1) + l4*cos(phi_4))^2 + l2^2 - l3^2)^2 + 4*l2^2*(l5 - l1*cos(phi_1) + l4*cos(phi_4))^2)^(1/2) - 2*l2*(l1*sin(phi_1) - l4*sin(phi_4)))/((l1*sin(phi_1) - l4*sin(phi_4))^2 + (l5 - l1*cos(phi_1) + l4*cos(phi_4))^2 + l2^2 - l3^2 + 2*l2*(l5 - l1*cos(phi_1) + l4*cos(phi_4)))))*(l2*sin(2*atan(((4*l2^2*(l1*sin(phi_1) - l4*sin(phi_4))^2 - ((l1*sin(phi_1) - l4*sin(phi_4))^2 + (l5 - l1*cos(phi_1) + l4*cos(phi_4))^2 + l2^2 - l3^2)^2 + 4*l2^2*(l5 - l1*cos(phi_1) + l4*cos(phi_4))^2)^(1/2) - 2*l2*(l1*sin(phi_1) - l4*sin(phi_4)))/((l1*sin(phi_1) - l4*sin(phi_4))^2 + (l5 - l1*cos(phi_1) + l4*cos(phi_4))^2 + l2^2 - l3^2 + 2*l2*(l5 - l1*cos(phi_1) + l4*cos(phi_4))))) + l1*sin(phi_1))*(((8*l2^2*l4*cos(phi_4)*(l1*sin(phi_1) - l4*sin(phi_4)) - 2*(2*l4*cos(phi_4)*(l1*sin(phi_1) - l4*sin(phi_4)) + 2*l4*sin(phi_4)*(l5 - l1*cos(phi_1) + l4*cos(phi_4)))*((l1*sin(phi_1) - l4*sin(phi_4))^2 + (l5 - l1*cos(phi_1) + l4*cos(phi_4))^2 + l2^2 - l3^2) + 8*l2^2*l4*sin(phi_4)*(l5 - l1*cos(phi_1) + l4*cos(phi_4)))/(2*(4*l2^2*(l1*sin(phi_1) - l4*sin(phi_4))^2 - ((l1*sin(phi_1) - l4*sin(phi_4))^2 + (l5 - l1*cos(phi_1) + l4*cos(phi_4))^2 + l2^2 - l3^2)^2 + 4*l2^2*(l5 - l1*cos(phi_1) + l4*cos(phi_4))^2)^(1/2)) - 2*l2*l4*cos(phi_4))/((l1*sin(phi_1) - l4*sin(phi_4))^2 + (l5 - l1*cos(phi_1) + l4*cos(phi_4))^2 + l2^2 - l3^2 + 2*l2*(l5 - l1*cos(phi_1) + l4*cos(phi_4))) - (((4*l2^2*(l1*sin(phi_1) - l4*sin(phi_4))^2 - ((l1*sin(phi_1) - l4*sin(phi_4))^2 + (l5 - l1*cos(phi_1) + l4*cos(phi_4))^2 + l2^2 - l3^2)^2 + 4*l2^2*(l5 - l1*cos(phi_1) + l4*cos(phi_4))^2)^(1/2) - 2*l2*(l1*sin(phi_1) - l4*sin(phi_4)))*(2*l2*l4*sin(phi_4) + 2*l4*cos(phi_4)*(l1*sin(phi_1) - l4*sin(phi_4)) + 2*l4*sin(phi_4)*(l5 - l1*cos(phi_1) + l4*cos(phi_4))))/((l1*sin(phi_1) - l4*sin(phi_4))^2 + (l5 - l1*cos(phi_1) + l4*cos(phi_4))^2 + l2^2 - l3^2 + 2*l2*(l5 - l1*cos(phi_1) + l4*cos(phi_4)))^2))/((((4*l2^2*(l1*sin(phi_1) - l4*sin(phi_4))^2 - ((l1*sin(phi_1) - l4*sin(phi_4))^2 + (l5 - l1*cos(phi_1) + l4*cos(phi_4))^2 + l2^2 - l3^2)^2 + 4*l2^2*(l5 - l1*cos(phi_1) + l4*cos(phi_4))^2)^(1/2) - 2*l2*(l1*sin(phi_1) - l4*sin(phi_4)))^2/((l1*sin(phi_1) - l4*sin(phi_4))^2 + (l5 - l1*cos(phi_1) + l4*cos(phi_4))^2 + l2^2 - l3^2 + 2*l2*(l5 - l1*cos(phi_1) + l4*cos(phi_4)))^2 + 1)*(l2*cos(2*atan(((4*l2^2*(l1*sin(phi_1) - l4*sin(phi_4))^2 - ((l1*sin(phi_1) - l4*sin(phi_4))^2 + (l5 - l1*cos(phi_1) + l4*cos(phi_4))^2 + l2^2 - l3^2)^2 + 4*l2^2*(l5 - l1*cos(phi_1) + l4*cos(phi_4))^2)^(1/2) - 2*l2*(l1*sin(phi_1) - l4*sin(phi_4)))/((l1*sin(phi_1) - l4*sin(phi_4))^2 + (l5 - l1*cos(phi_1) + l4*cos(phi_4))^2 + l2^2 - l3^2 + 2*l2*(l5 - l1*cos(phi_1) + l4*cos(phi_4))))) - l5/2 + l1*cos(phi_1))^2)))/((l2*sin(2*atan(((4*l2^2*(l1*sin(phi_1) - l4*sin(phi_4))^2 - ((l1*sin(phi_1) - l4*sin(phi_4))^2 + (l5 - l1*cos(phi_1) + l4*cos(phi_4))^2 + l2^2 - l3^2)^2 + 4*l2^2*(l5 - l1*cos(phi_1) + l4*cos(phi_4))^2)^(1/2) - 2*l2*(l1*sin(phi_1) - l4*sin(phi_4)))/((l1*sin(phi_1) - l4*sin(phi_4))^2 + (l5 - l1*cos(phi_1) + l4*cos(phi_4))^2 + l2^2 - l3^2 + 2*l2*(l5 - l1*cos(phi_1) + l4*cos(phi_4))))) + l1*sin(phi_1))^2/(l2*cos(2*atan(((4*l2^2*(l1*sin(phi_1) - l4*sin(phi_4))^2 - ((l1*sin(phi_1) - l4*sin(phi_4))^2 + (l5 - l1*cos(phi_1) + l4*cos(phi_4))^2 + l2^2 - l3^2)^2 + 4*l2^2*(l5 - l1*cos(phi_1) + l4*cos(phi_4))^2)^(1/2) - 2*l2*(l1*sin(phi_1) - l4*sin(phi_4)))/((l1*sin(phi_1) - l4*sin(phi_4))^2 + (l5 - l1*cos(phi_1) + l4*cos(phi_4))^2 + l2^2 - l3^2 + 2*l2*(l5 - l1*cos(phi_1) + l4*cos(phi_4))))) - l5/2 + l1*cos(phi_1))^2 + 1);
end
